simulink model "ajay"  (R2024b)
settings: Solver=ode45  StartTime=0.0  StopTime=75  RelTol=1e-3  EnableMultiTasking=on
PreLoadFcn:
  | load asbSkyHoggData.mat
StopFcn:
  | open_system('asbSkyHogg/Vehicle System Model/Avionics/Autopilot/Altitude')
model workspace (MAT data in the model file):
  LatLong0 = [45 120]
  Sref = 20.9775
  Tc = 0.0166666666667
  Thrust = 2512.574
  Ts = 0
  V0 = 93.1047999839
  alpha0 = 0.0170924
  alt0 = 2000
  beta0 = 0
  bref = 12.5425
  cbar = 1.7526
  cg_0 = [2.158 0 0]
  g_0 = [0 0 9.81]
  heading0 = 0
  inertia = [5787.969  0  117.64; 0  6928.93  0; -117.64  0  11578.329]
  mass = 1299.21378662
  maxdef_aileron = 30
  maxdef_elevator = 20
  maxdef_rudder = 60
  mindef_aileron = -30
  mindef_elevator = -20
  mindef_rudder = -60
  mpoperpoint = []
  theta0 = 0.017092
  wn_act = 44
  wy0 = 0
  z_act = 0.7
undefined symbols (not defined in the file): Earth, F, Light, MIL, pa28, statdyn, WGS84
libraries: aerolibasang x4, aerolibwind2 x3, aerolibtransform2 x3, aerolibactuator x3, aerolibatmos2 x2, aerolibconvert2 x2, aerolibadyn x2, aerolibfltsims x2, simulink x1, simulink_extras x1, aerolibnav x1, sharedtransform x1
Description:
  | Lightweight Airplane Design
  | 
  | This is the three degree-of-freedom model of a lightweight four-seater
  | low wing monoplane with a longitudinal autopilot.
settings Model: Creator=The MathWorks, Inc.  LastModifiedBy=91964
settings SolverCC: AlgebraicLoopSolver=TrustRegion  MaxZcPerStep=1
settings DataIOCC: ExternalInput=getinputstruct(op_skyhogg3dof2V5)  InitialState=getstatestruct(op_skyhogg3dof2V5)  LimitDataPoints=on  SaveFormat=Array  ReturnWorkspaceOutputs=off
settings OptimizationCC: ExpressionDepthLimit=2147483647  InitFltsAndDblsToZero=on  LifeSpan=inf
settings DebuggingCC: WriteAfterWriteMsg=DisableAll  AlgebraicLoopMsg=none  SaveWithParameterizedLinksMsg=none  SignalResolutionControl=TryResolveAllWithWarning  FcnCallInpInsideContextMsg=warning  UniqueDataStoreMsg=error  AllowSymbolicDim=off  StateNameClashWarn=warning  SubsystemReferenceDiagnosticForUnitTest=warning  StrictBusMsg=ErrorOnBusTreatedAsVector  SFUnexpectedBacktrackingDiag=warning  SFNoUnconditionalDefaultTransitionDiag=warning  SFExecutionAtInitializationDiag=none  ArithmeticOperatorsInVariantConditions=warning
settings HardwareCC: ProdBitPerPointer=32  ProdBitPerSizeT=32  ProdBitPerPtrDiffT=32  ProdLargestAtomicFloat=None  ProdIntDivRoundTo=Undefined  ProdEndianess=Unspecified  ProdWordSize=32  ProdHWDeviceType=32-bit Generic
settings ModelReferenceCC: EnableRefExpFcnMdlSchedulingChecks=on  PropagateSignalLabelsOutOfModel=off
settings SFSimCC: SimUseLocalCustomCode=off  CustomCodeUndefinedFunction=UseInterfaceOnly
settings RTWCC: RTWUseLocalCustomCode=off  GPUComputeCapability=3.5  DLArmComputeVersion=19.05
settings CodeAppCC: StateflowObjectComments=on
settings GRTTargetCC: TargetFcnLib=ansi_tfl_tmw.mat  TargetLangStandard=C89/C90 (ANSI)  CombineOutputUpdateFcns=off  GRTInterface=on
settings ConfigComp: CovMetricSettings=dw  CovSaveCumulativeToWorkspaceVar=on  CovSaveSingleToWorkspaceVar=on  CovExternalEMLEnable=off  CovSFcnEnable=off

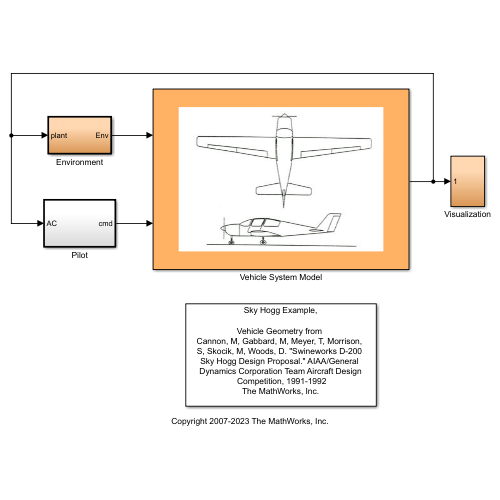
[thumbnail: Simulink's stored preview of the top-level diagram]
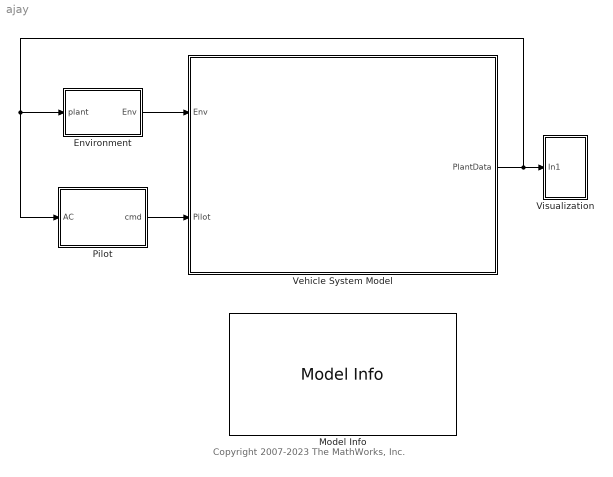
== system ajay ==
  note: Copyright 2007-2023 The MathWorks, Inc.
  Environment : Subsystem  TreatAsAtomicUnit=on
  Model Info : simulink/Model-Wide Utilities/Model Info  Frame=on  DisplayStringWithTags=|  HorizontalTextAlignment=Center  LeftAlignmentValue=0.5
      | Sky Hogg Example,
      | 
      | Vehicle Geometry from 
      | Cannon, M, Gabbard, M, Meyer, T, Morrison, 
      | S, Skocik, M, Woods, D. "Swineworks D-200 
      | Sky Hogg Design Proposal." AIAA/General 
      | Dynamics Corporation Team Aircraft Design
      |  Competition, 1991-1992
      | %<Creator>
      | %<ModifiedComment>
  Pilot : Subsystem  TreatAsAtomicUnit=on
  Vehicle System Model : Subsystem
      mask Display: image('asbSkyHogg.jpg',[.1 .1 .8 .8],'on')
  Visualization : Subsystem
  wires:
  Environment/1(Env) -> Vehicle System Model/1(Env)
  Vehicle System Model/1(PlantData) -> Environment/1(plant), Pilot/1(AC), Visualization/1(In1)
  Pilot/1(cmd) -> Vehicle System Model/2(Pilot)

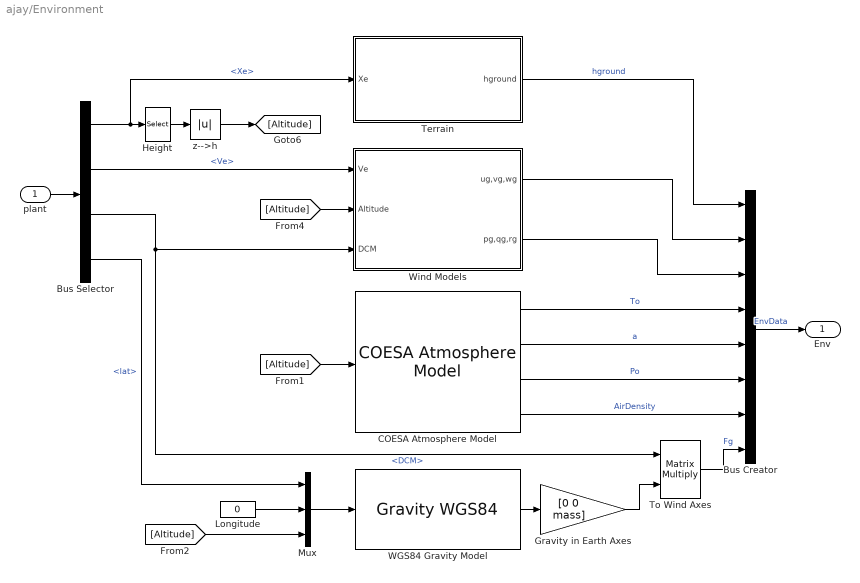
== system ajay/Environment ==
  plant : Inport
  Bus Creator : BusCreator  Inputs='hground','WindVelocity','WindAngularRates','To','a','Po','AirDensity','Fg'
  Bus Selector : BusSelector  OutputSignals=Xe,Ve,DCM,lat
  COESA Atmosphere Model : aerolibatmos2/COESA Atmosphere Model  units=Metric (MKS)  spec=1976 COESA-extended U.S. Standard Atmosphere  model=Profile  profile_var=High temperature  profile_percent=1%  profile_alt=5 km (16404 ft)  envelope_var=High temperature  envelope_percent=1%  action=Warning
  Gravity in Earth Axes : Gain  Gain=[0 0 mass]  SaturateOnIntegerOverflow=on  OutDataTypeStr=Inherit: Same as input  ParamDataTypeStr=Inherit: Same as input
  Height : Selector  IndexMode=Zero-based  InputPortWidth=3  IndexOptions=Index vector (dialog)  Indices=2  OutputSizes=1
  Longitude : Constant  Value=0
  Mux : Mux  Inputs=3
  Terrain : Subsystem
  To Wind Axes : Product  Multiplication=Matrix(*)  InputSameDT=on  SaturateOnIntegerOverflow=on  OutDataTypeStr=Inherit: Same as first input
  "WGS84 Gravity Model  " : GravityWGS84
  Wind Models : Subsystem
  z-->h : Abs
  Env : Outport  InitialOutput=0  VectorParamsAs1DForOutWhenUnconnected=off
  wires:
  Bus Selector/3 -> To Wind Axes/1, Wind Models/3(DCM)  "<DCM>"
  Bus Selector/2 -> Wind Models/1(Ve)  "<Ve>"
  Bus Selector/1 -> Height/1, Terrain/1(Xe)  "<Xe>"
  [Altitude] -> COESA Atmosphere Model/1
  [Altitude] -> Mux/3
  [Altitude] -> Wind Models/2(Altitude)
  z-->h/1 -> [Altitude]
  plant/1 -> Bus Selector/1
  Bus Creator/1 -> Env/1  "EnvData"
  To Wind Axes/1 -> Bus Creator/8  "Fg"
  Gravity in Earth Axes/1 -> To Wind Axes/2
  "WGS84 Gravity Model  "/1 -> Gravity in Earth Axes/1
  Bus Selector/4 -> Mux/1  "<lat>"
  Height/1 -> z-->h/1
  COESA Atmosphere Model/1 -> Bus Creator/4  "To"
  COESA Atmosphere Model/3 -> Bus Creator/6  "Po"
  COESA Atmosphere Model/2 -> Bus Creator/5  "a"
  COESA Atmosphere Model/4 -> Bus Creator/7  "AirDensity"
  Wind Models/2(pg,qg,rg) -> Bus Creator/3
  Wind Models/1(ug,vg,wg) -> Bus Creator/2
  Terrain/1(hground) -> Bus Creator/1  "hground"
  Mux/1 -> "WGS84 Gravity Model  "/1
  Longitude/1 -> Mux/2

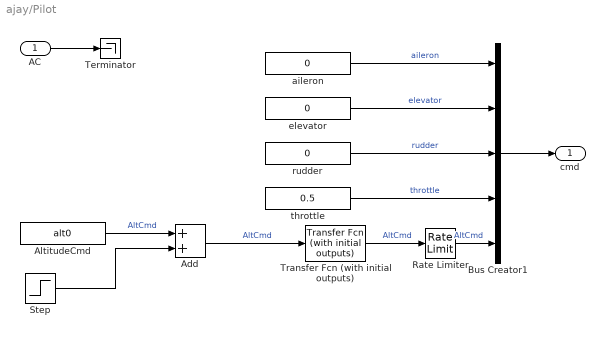
== system ajay/Pilot ==
  AC : Inport
  Add : Sum
  AltitudeCmd : Constant  Value=alt0  OutDataTypeStr=double
  Bus Creator1 : BusCreator  Inputs=5
  Rate Limiter : RateLimiter  RisingSlewLimit=500/3/60  SampleTimeMode=inherited  InitialCondition=2000
  Step : Step  Time=5  After=50  SampleTime=0
  Terminator : Terminator
  Transfer Fcn (with initial outputs) : simulink_extras/Additional Linear/Transfer Fcn (with initial outputs)  N=.25  D=[1,.25]  Y0=2000  U0=2000
  aileron : Constant  Value=0  OutDataTypeStr=single
  elevator : Constant  Value=0  OutDataTypeStr=single
  rudder : Constant  Value=0  OutDataTypeStr=single
  throttle : Constant  Value=0.5  OutDataTypeStr=double
  cmd : Outport  VectorParamsAs1DForOutWhenUnconnected=off
  wires:
  elevator/1 -> Bus Creator1/2  "elevator"
  aileron/1 -> Bus Creator1/1  "aileron"
  throttle/1 -> Bus Creator1/4  "throttle"
  rudder/1 -> Bus Creator1/3  "rudder"
  Bus Creator1/1 -> cmd/1
  AC/1 -> Terminator/1
  AltitudeCmd/1 -> Add/1  "AltCmd"
  Step/1 -> Add/2
  Add/1 -> Transfer Fcn (with initial outputs)/1  "AltCmd"
  Rate Limiter/1 -> Bus Creator1/5  "AltCmd"
  Transfer Fcn (with initial outputs)/1 -> Rate Limiter/1  "AltCmd"

== system ajay/Vehicle System Model ==
  Env : Inport
  Pilot : Inport  Port=2
  Avionics : Subsystem
  "Env " : InportShadow
  Flight Sensors : Subsystem
  "Pilot " : InportShadow  Port=2
  Vehicle : Subsystem
  PlantData : Outport  VectorParamsAs1DForOutWhenUnconnected=off
  wires:
  Env/1 -> Vehicle/1(Env)
  Vehicle/1(PlantData) -> PlantData/1, Avionics/1(PlantData), Flight Sensors/2(plant)
  Flight Sensors/1(sensed) -> Avionics/2(Sensors)
  Avionics/1(ActCmd) -> Vehicle/2(ActCmd)
  Pilot/1 -> Vehicle/3(Pilot)
  "Env "/1 -> Flight Sensors/1(Env)
  "Pilot "/1 -> Avionics/3(Pilot)

== system ajay/Visualization ==
  note: For FlightGear visualization only, we use the model for Piper Cherokee Warrior II.
  note: 3. To start FlightGear, generate run script and run generated batch file by typing
      |      dos('runfg.bat &') at the MATLAB command line.
  note: 1. See the Aerospace Blockset User's Guide for instructions to set up FlightGear.
  note: 2. Install the pa28-161 geometry model to FlightGear's data/Aircraft
      |     directory. The geometry is downloadable from www.flightgear.org.
  In1 : Inport
  Bus Selector1 : BusSelector  OutputSignals=long,lat,alt,body angles
  Bus to Vector3 : BusToVector
  FlightGear Preconfigured 6DoF Animation : aerolibfltsims/FlightGear Preconfigured 6DoF Animation  xFlightGearVersion=v2019.1  DestinationIpAddress=127.0.0.1  DestinationPort=5502  SampleTime=1/30  packetVersion=24
  Generate Run Script (if FG is installed) : aerolibfltsims/Generate Run Script  Architecture=Default  dataFlow=Send  GeometryModelName=pa28-161  AirportId=KSFO  RunwayId=10L  InitialAltitude=7224  InitialHeading=113  OffsetDistance=4.72  OffsetAzimuth=0  InstallScenery=on  DisableShaders=on  OriginAddress=127.0.0.1  DestinationPort=5502  OriginPort=5505  LocalAddress=127.0.0.1  OutputFileName=runfg.bat  FlightGearBaseDirectory=C:\Program Files\FlightGear
  Mux1 : Mux
  wires:
  In1/1 -> Bus Selector1/1
  Bus Selector1/1 -> Mux1/1  "<long>"
  Bus Selector1/2 -> Mux1/2  "<lat>"
  Bus Selector1/3 -> Mux1/3  "<alt>"
  Bus Selector1/4 -> Bus to Vector3/1  "<body angles>"
  Mux1/1 -> FlightGear Preconfigured 6DoF Animation/1
  Bus to Vector3/1 -> Mux1/4

== system ajay/Environment/Terrain ==
  note: This part of the system defines the interface for the terrain model that will be developed in detail later on.
  Xe : Inport
  Terminator : Terminator
  hground_value : Constant  Value=0  OutDataTypeStr=single
  hground : Outport  Unit=m  VectorParamsAs1DForOutWhenUnconnected=off
  wires:
  hground_value/1 -> hground/1  "hground"
  Xe/1 -> Terminator/1

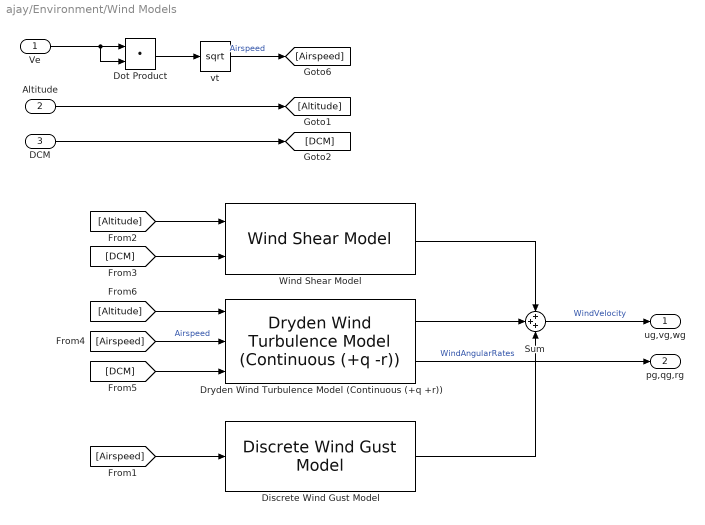
== system ajay/Environment/Wind Models ==
  Ve : Inport
  Altitude : Inport  Port=2
  DCM : Inport  Port=3
  Discrete Wind Gust Model : aerolibwind2/Discrete Wind Gust Model  units=Metric (MKS)  Gx=off  Gy=off  Gz=off  t_0=20  d_m=[120 120 80]  v_m=[3.5 3.0 3.0]
  Dot Product : DotProduct  InputSameDT=off  OutDataTypeStr=Inherit: Inherit via internal rule
  Dryden Wind Turbulence Model (Continuous (+q +r)) : aerolibwind2/Dryden Wind Turbulence Model  (Continuous (+q -r))  units=Metric (MKS)  spec=MIL-F-8785C  model=Continuous Dryden (+q +r)  W20=5  Wdeg=0  TurbProb=10^-2 - Light  L_high=533.4  Wingspan=4  ts=0.1  Seed=[23341 23342 23343 23344]  T_on=off
  Sum : Sum  Inputs=+++  InputSameDT=on  SaturateOnIntegerOverflow=on  OutDataTypeStr=Inherit: Same as first input
  Wind Shear Model : aerolibwind2/Wind Shear Model  units=Metric (MKS)  phase=Category C - Terminal Flight Phase  W_20=1  Wdeg=0
  vt : Sqrt
  ug,vg,wg : Outport  Unit=m/s  VectorParamsAs1DForOutWhenUnconnected=off
  pg,qg,rg : Outport  Port=2  Unit=rad/second  VectorParamsAs1DForOutWhenUnconnected=off
  wires:
  [Altitude] -> Dryden Wind Turbulence Model (Continuous (+q +r))/1
  [DCM] -> Dryden Wind Turbulence Model (Continuous (+q +r))/3
  [DCM] -> Wind Shear Model/2
  DCM/1 -> [DCM]
  [Altitude] -> Wind Shear Model/1
  Altitude/1 -> [Altitude]
  [Airspeed] -> Discrete Wind Gust Model/1
  vt/1 -> [Airspeed]  "Airspeed"
  Dot Product/1 -> vt/1
  Dryden Wind Turbulence Model (Continuous (+q +r))/2 -> pg,qg,rg/1  "WindAngularRates"
  [Airspeed] -> Dryden Wind Turbulence Model (Continuous (+q +r))/2  "Airspeed"
  Sum/1 -> ug,vg,wg/1  "WindVelocity"
  Discrete Wind Gust Model/1 -> Sum/3
  Dryden Wind Turbulence Model (Continuous (+q +r))/1 -> Sum/2
  Wind Shear Model/1 -> Sum/1
  Ve/1 -> Dot Product/2, Dot Product/1

== system ajay/Vehicle System Model/Avionics ==
  PlantData : Inport
  Sensors : Inport  Port=2
  Pilot : Inport  Port=3
  Air Data Computer : Subsystem  TreatAsAtomicUnit=on
  Autopilot : Subsystem
  Bus Creator : BusCreator  Inputs=2
  Bus Selector1 : BusSelector  OutputSignals=Ab,w,wdot
  Center of Gravity : Constant  Value=cg_0  SampleTime=Tc
  Gravity (not in Accels) : Constant  Value=g_0  SampleTime=Tc
  Guidance : Subsystem
  Three-axis IMU : aerolibnav/Three-axis Inertial Measurement Unit  units=Metric (MKS)  imu=cg_0  i_Ts=Tc  dtype_a=off  w_a=190  z_a=0.707  a_sf_cc=[1 0 0; 0 1 0; 0 0 1]  a_bias=[0 0 0]  a_sat="[-inf  -inf  -inf  inf inf inf]"  dtype_g=off  w_g=190  z_g=0.707  g_sf_cc=[1 0 0; 0 1 0; 0 0 1]  g_bias=[0 0 0]  g_sens=[0 0 0]  g_sat="[-inf  -inf  -inf  inf inf inf]"  i_rand=off  i_seeds=[23093 23094 23095 23096 23097 23098]  i_pow=[0.001 0.001 0.001 0.0001 0.0001 0.0001]
  ActCmd : Outport  VectorParamsAs1DForOutWhenUnconnected=off
  wires:
  Three-axis IMU/2 -> Bus Creator/2
  Three-axis IMU/1 -> Bus Creator/1
  Bus Selector1/1 -> Three-axis IMU/1  "<Ab>"
  Center of Gravity/1 -> Three-axis IMU/4
  Bus Creator/1 -> Autopilot/1(AvionicBus), Guidance/2(AvionicBus)
  PlantData/1 -> Bus Selector1/1
  Bus Selector1/2 -> Three-axis IMU/2  "<w>"
  Bus Selector1/3 -> Three-axis IMU/3  "<wdot>"
  Gravity (not in Accels)/1 -> Three-axis IMU/5
  Sensors/1 -> Air Data Computer/1(sensors)
  Autopilot/1(cmd) -> ActCmd/1
  Air Data Computer/1(AirData) -> Autopilot/2(AirData), Guidance/1(AirData)
  Guidance/1(cmd) -> Autopilot/3(guidance)
  Pilot/1 -> Guidance/3(Pilot)

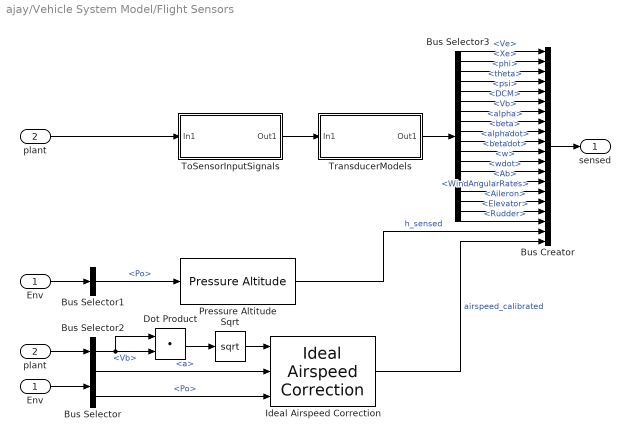
== system ajay/Vehicle System Model/Flight Sensors ==
  Env : Inport
  plant : Inport  Port=2
  Bus Creator : BusCreator  Inputs=20
  Bus Selector : BusSelector  OutputSignals=a,Po
  Bus Selector1 : BusSelector  OutputSignals=Po
  Bus Selector2 : BusSelector  OutputSignals=Vb
  Bus Selector3 : BusSelector  OutputSignals=Ve,Xe,body angles.phi,body angles.theta,body angles.psi,DCM,Vb,alpha,beta,alphadot,betadot,w,wdot,Ab,WindAngularRates,Act_positions.Aileron,Act_positions.Elevator,Act_positions.Rudder
  Dot Product : DotProduct  OutDataTypeStr=Inherit: Inherit via internal rule
  "Env " : InportShadow
  Ideal Airspeed Correction : aerolibasang/Ideal Airspeed Correction  units=Metric (MKS)  vel_in=TAS  vel_out_tas=CAS  vel_out_eas=CAS  vel_out_cas=TAS  method=Table Lookup  SubOnly=off  action=Error
  Pressure Altitude : aerolibatmos2/Pressure Altitude  units=Metric (MKS)  action=Warning
  Sqrt : Sqrt
  ToSensorInputSignals : Subsystem
  TransducerModels : Subsystem
  "plant " : InportShadow  Port=2
  sensed : Outport  VectorParamsAs1DForOutWhenUnconnected=off
  wires:
  ToSensorInputSignals/1(Out1) -> TransducerModels/1(In1)
  Env/1 -> Bus Selector/1
  TransducerModels/1(Out1) -> Bus Selector3/1
  plant/1 -> ToSensorInputSignals/1(In1)
  Bus Selector/1 -> Ideal Airspeed Correction/2  "<a>"
  Bus Selector/2 -> Ideal Airspeed Correction/3  "<Po>"
  Bus Selector1/1 -> Pressure Altitude/1  "<Po>"
  "Env "/1 -> Bus Selector1/1
  "plant "/1 -> Bus Selector2/1
  Dot Product/1 -> Sqrt/1
  Sqrt/1 -> Ideal Airspeed Correction/1
  Bus Selector2/1 -> Dot Product/2, Dot Product/1  "<Vb>"
  Bus Selector3/1 -> Bus Creator/1  "<Ve>"
  Bus Selector3/2 -> Bus Creator/2  "<Xe>"
  Bus Selector3/3 -> Bus Creator/3  "<phi>"
  Bus Selector3/4 -> Bus Creator/4  "<theta>"
  Bus Selector3/5 -> Bus Creator/5  "<psi>"
  Bus Selector3/6 -> Bus Creator/6  "<DCM>"
  Bus Selector3/7 -> Bus Creator/7  "<Vb>"
  Bus Selector3/8 -> Bus Creator/8  "<alpha>"
  Bus Selector3/9 -> Bus Creator/9  "<beta>"
  Bus Selector3/10 -> Bus Creator/10  "<alphadot>"
  Bus Selector3/11 -> Bus Creator/11  "<betadot>"
  Bus Selector3/12 -> Bus Creator/12  "<w>"
  Bus Selector3/13 -> Bus Creator/13  "<wdot>"
  Bus Selector3/14 -> Bus Creator/14  "<Ab>"
  Bus Creator/1 -> sensed/1
  Bus Selector3/15 -> Bus Creator/15  "<WindAngularRates>"
  Bus Selector3/16 -> Bus Creator/16  "<Aileron>"
  Bus Selector3/17 -> Bus Creator/17  "<Elevator>"
  Bus Selector3/18 -> Bus Creator/18  "<Rudder>"
  Pressure Altitude/1 -> Bus Creator/19  "h_sensed"
  Ideal Airspeed Correction/1 -> Bus Creator/20  "airspeed_calibrated"

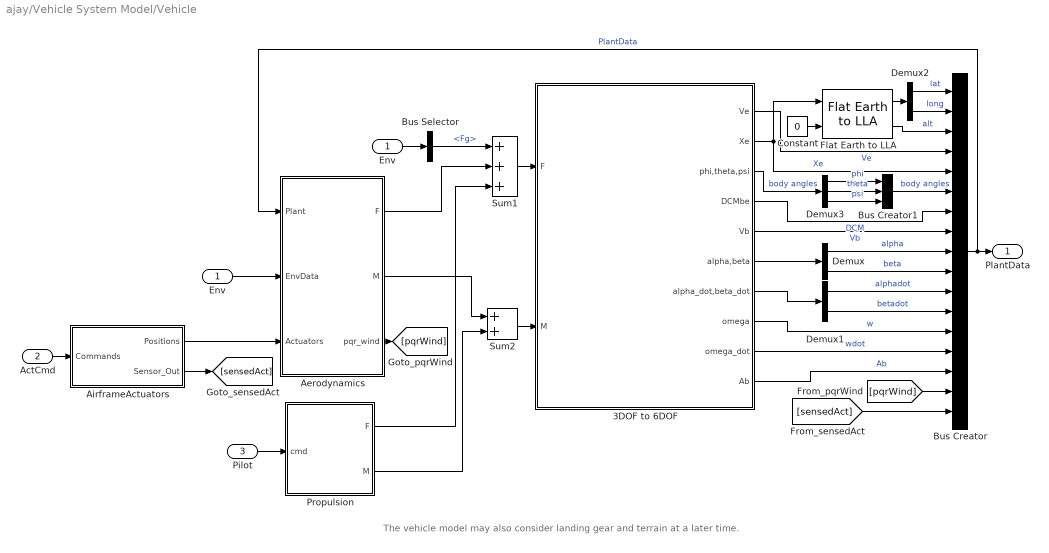
== system ajay/Vehicle System Model/Vehicle ==
  note: The vehicle model may also consider landing gear and terrain at a later time.
  Env : Inport
  ActCmd : Inport  Port=2
  Pilot : Inport  Port=3
  3DOF to 6DOF : Subsystem
  Aerodynamics : Subsystem
  AirframeActuators : Subsystem
  Bus Creator : BusCreator  Inputs=17
  Bus Creator1 : BusCreator  Inputs=3
  Bus Selector : BusSelector  OutputSignals=Fg
  Constant : Constant  Value=0
  Demux : Demux  Outputs=2
  Demux1 : Demux  Outputs=2
  Demux2 : Demux  Outputs=2
  Demux3 : Demux  Outputs=3
  "Env " : InportShadow
  Flat Earth to LLA : aerolibtransform2/Flat Earth to LLA  units=Metric (MKS)  ptype=Earth (WGS84)  F=1/298.257223563  R=6378137  refPosPort=off  LL0=LatLong0  psi=heading0
  Propulsion : Subsystem
      settings: RTWSystemCode=Inline
  Sum1 : Sum  Inputs=+++  InputSameDT=on  SaturateOnIntegerOverflow=on  OutDataTypeStr=Inherit: Same as first input
  Sum2 : Sum  InputSameDT=on  SaturateOnIntegerOverflow=on  OutDataTypeStr=Inherit: Same as first input
  PlantData : Outport  VectorParamsAs1DForOutWhenUnconnected=off
  wires:
  Sum1/1 -> 3DOF to 6DOF/1(F)
  Sum2/1 -> 3DOF to 6DOF/2(M)
  3DOF to 6DOF/3(phi,theta,psi) -> Demux3/1  "body angles"
  3DOF to 6DOF/4(DCMbe) -> Bus Creator/7  "DCM"
  3DOF to 6DOF/5(Vb) -> Bus Creator/8  "Vb"
  3DOF to 6DOF/6(alpha,beta) -> Demux/1
  3DOF to 6DOF/7(alpha_dot,beta_dot) -> Demux1/1
  3DOF to 6DOF/9(omega_dot) -> Bus Creator/14  "wdot"
  3DOF to 6DOF/10(Ab) -> Bus Creator/15  "Ab"
  Aerodynamics/1(F) -> Sum1/2
  Aerodynamics/2(M) -> Sum2/1
  Propulsion/1(F) -> Sum1/3
  Propulsion/2(M) -> Sum2/2
  Bus Selector/1 -> Sum1/1  "<Fg>"
  Env/1 -> Aerodynamics/2(EnvData)
  ActCmd/1 -> AirframeActuators/1(Commands)
  Pilot/1 -> Propulsion/1(cmd)
  "Env "/1 -> Bus Selector/1
  AirframeActuators/1(Positions) -> Aerodynamics/3(Actuators)
  Aerodynamics/3(pqr_wind) -> [pqrWind]
  [pqrWind] -> Bus Creator/16
  AirframeActuators/2(Sensor_Out) -> [sensedAct]
  [sensedAct] -> Bus Creator/17
  Constant/1 -> Flat Earth to LLA/2
  Flat Earth to LLA/2 -> Bus Creator/3  "alt"
  Flat Earth to LLA/1 -> Demux2/1
  Demux2/1 -> Bus Creator/1  "lat"
  Demux2/2 -> Bus Creator/2  "long"
  Demux1/1 -> Bus Creator/11  "alphadot"
  Demux1/2 -> Bus Creator/12  "betadot"
  Demux3/1 -> Bus Creator1/1  "phi"
  Demux3/2 -> Bus Creator1/2  "theta"
  Demux3/3 -> Bus Creator1/3  "psi"
  Bus Creator1/1 -> Bus Creator/6  "body angles"
  3DOF to 6DOF/8(omega) -> Bus Creator/13  "w"
  Demux/2 -> Bus Creator/10  "beta"
  Demux/1 -> Bus Creator/9  "alpha"
  3DOF to 6DOF/1(Ve) -> Bus Creator/4  "Ve"
  3DOF to 6DOF/2(Xe) -> Flat Earth to LLA/1, Bus Creator/5  "Xe"
  Bus Creator/1 -> Aerodynamics/1(Plant), PlantData/1  "PlantData"

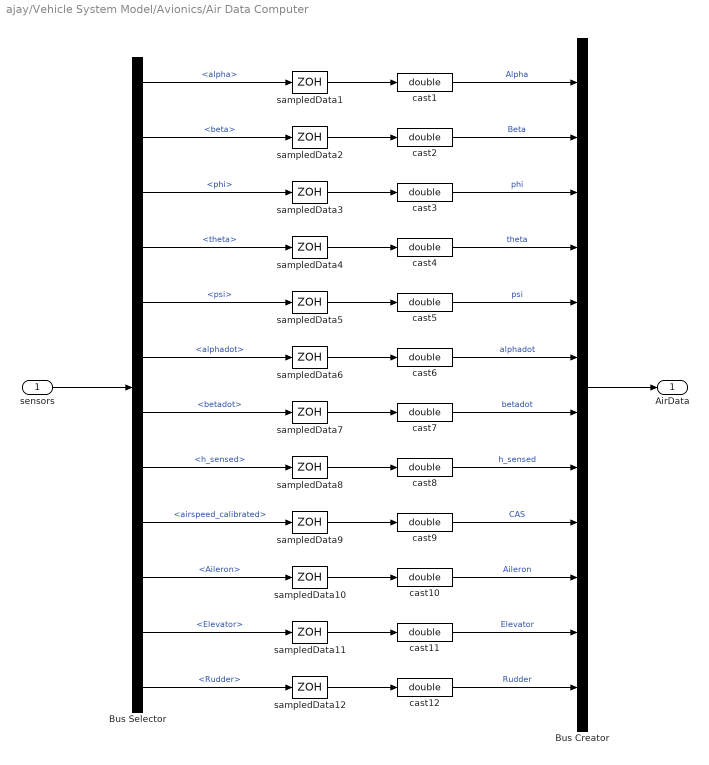
== system ajay/Vehicle System Model/Avionics/Air Data Computer ==
  sensors : Inport  SampleTime=Ts
  Bus Creator : BusCreator  Inputs=12
  Bus Selector : BusSelector  OutputSignals=alpha,beta,phi,theta,psi,alphadot,betadot,h_sensed,airspeed_calibrated,Aileron,Elevator,Rudder
  cast{1..12} (12 alike) : DataTypeConversion  OutDataTypeStr=double  SaturateOnIntegerOverflow=off  RndMeth=Floor
  sampledData{1..12} (12 alike) : ZeroOrderHold  SampleTime=Tc
  AirData : Outport  VectorParamsAs1DForOutWhenUnconnected=off
  wires:
  sensors/1 -> Bus Selector/1
  Bus Creator/1 -> AirData/1
  cast1/1 -> Bus Creator/1  "Alpha"
  cast2/1 -> Bus Creator/2  "Beta"
  cast3/1 -> Bus Creator/3  "phi"
  cast12/1 -> Bus Creator/12  "Rudder"
  cast10/1 -> Bus Creator/10  "Aileron"
  cast9/1 -> Bus Creator/9  "CAS"
  cast8/1 -> Bus Creator/8  "h_sensed"
  cast7/1 -> Bus Creator/7  "betadot"
  cast6/1 -> Bus Creator/6  "alphadot"
  cast5/1 -> Bus Creator/5  "psi"
  sampledData1/1 -> cast1/1
  sampledData2/1 -> cast2/1
  sampledData3/1 -> cast3/1
  sampledData4/1 -> cast4/1
  sampledData5/1 -> cast5/1
  sampledData6/1 -> cast6/1
  sampledData7/1 -> cast7/1
  sampledData8/1 -> cast8/1
  sampledData9/1 -> cast9/1
  sampledData10/1 -> cast10/1
  cast4/1 -> Bus Creator/4  "theta"
  Bus Selector/1 -> sampledData1/1  "<alpha>"
  Bus Selector/2 -> sampledData2/1  "<beta>"
  Bus Selector/3 -> sampledData3/1  "<phi>"
  Bus Selector/4 -> sampledData4/1  "<theta>"
  Bus Selector/5 -> sampledData5/1  "<psi>"
  Bus Selector/6 -> sampledData6/1  "<alphadot>"
  Bus Selector/7 -> sampledData7/1  "<betadot>"
  Bus Selector/8 -> sampledData8/1  "<h_sensed>"
  Bus Selector/9 -> sampledData9/1  "<airspeed_calibrated>"
  Bus Selector/10 -> sampledData10/1  "<Aileron>"
  Bus Selector/12 -> sampledData12/1  "<Rudder>"
  sampledData11/1 -> cast11/1
  sampledData12/1 -> cast12/1
  Bus Selector/11 -> sampledData11/1  "<Elevator>"
  cast11/1 -> Bus Creator/11  "Elevator"

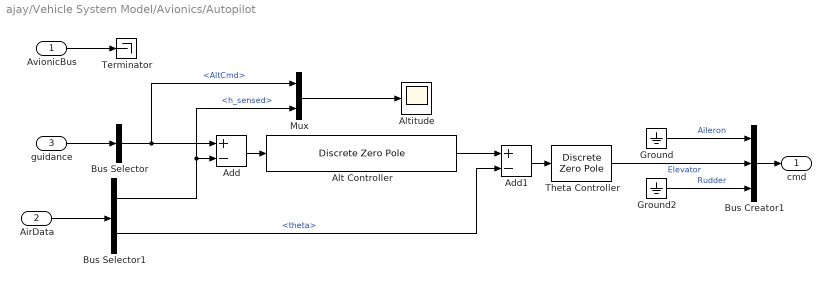
== system ajay/Vehicle System Model/Avionics/Autopilot ==
  AvionicBus : Inport
  AirData : Inport  Port=2
  guidance : Inport  Port=3
  Add : Sum  Inputs=+-
  Add1 : Sum  Inputs=+-
  Alt Controller : DiscreteZeroPole  Zeros=[0.998853192323097;0.977076159863424]  Poles=[1;0.920841826994512]  Gain=0.0337283240400683  SampleTime=Tc
  Altitude : Scope
  Bus Creator1 : BusCreator  Inputs=3
  Bus Selector : BusSelector  OutputSignals=AltCmd
  Bus Selector1 : BusSelector  OutputSignals=h_sensed,theta
  Ground : Ground
  Ground2 : Ground
  Mux : Mux  Inputs=2
  Terminator : Terminator
  Theta Controller : DiscreteZeroPole  Zeros=0.999268009521977  Poles=1  Gain=-261.8699347622  SampleTime=Tc
  cmd : Outport  VectorParamsAs1DForOutWhenUnconnected=off
  wires:
  Add1/1 -> Theta Controller/1
  Alt Controller/1 -> Add1/1
  Add/1 -> Alt Controller/1
  Bus Selector/1 -> Mux/1, Add/1  "<AltCmd>"
  guidance/1 -> Bus Selector/1
  AirData/1 -> Bus Selector1/1
  AvionicBus/1 -> Terminator/1
  Bus Creator1/1 -> cmd/1
  Ground2/1 -> Bus Creator1/3  "Rudder"
  Theta Controller/1 -> Bus Creator1/2  "Elevator"
  Ground/1 -> Bus Creator1/1  "Aileron"
  Mux/1 -> Altitude/1
  Bus Selector1/1 -> Mux/2, Add/2  "<h_sensed>"
  Bus Selector1/2 -> Add1/2  "<theta>"

== system ajay/Vehicle System Model/Avionics/Guidance ==
  note: This part of the system defines the interface for the guidance model that will be developed in detail later on.
  AirData : Inport
  AvionicBus : Inport  Port=2
  Pilot : Inport  Port=3
  Bus Creator1 : BusCreator  Inputs=2
  Bus Selector : BusSelector  OutputSignals=AltCmd
  Ground1 : Ground
  Terminator : Terminator
  Terminator1 : Terminator
  cmd : Outport  VectorParamsAs1DForOutWhenUnconnected=off
  wires:
  Pilot/1 -> Bus Selector/1
  Bus Selector/1 -> Bus Creator1/1  "<AltCmd>"
  Ground1/1 -> Bus Creator1/2  "Elevator angle"
  Bus Creator1/1 -> cmd/1
  AvionicBus/1 -> Terminator/1
  AirData/1 -> Terminator1/1

== system ajay/Vehicle System Model/Flight Sensors/ToSensorInputSignals ==
  note: This part of the system defines the interface for the measurement noise model that
      |  will be developed in detail later on.
  In1 : Inport
  Out1 : Outport  VectorParamsAs1DForOutWhenUnconnected=off
  wires:
  In1/1 -> Out1/1

== system ajay/Vehicle System Model/Flight Sensors/TransducerModels ==
  note: This part of the system defines the interface for the transducers model that
      |  will be developed in detail later on.
  In1 : Inport
  Out1 : Outport  VectorParamsAs1DForOutWhenUnconnected=off
  wires:
  In1/1 -> Out1/1

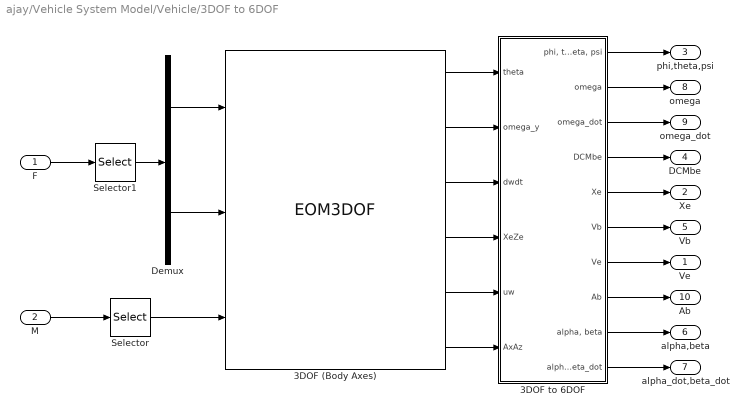
== system ajay/Vehicle System Model/Vehicle/3DOF to 6DOF ==
  F : Inport
  M : Inport  Port=2
  3DOF (Body Axes) : EOM3DOF  v_ini=V0  theta_ini=theta0  q_ini=wy0  alpha_ini=alpha0  pos_ini=[0 -alt0]  mass=mass  Iyy=inertia(2,2)  g=0  mdot_flag=off
  3DOF to 6DOF : Subsystem
  Demux : Demux  Outputs=2
  Selector : Selector  IndexMode=Zero-based  InputPortWidth=3  IndexOptions=Index vector (dialog)  Indices=1  OutputSizes=1
  Selector1 : Selector  IndexMode=Zero-based  InputPortWidth=3  IndexOptions=Index vector (dialog)  Indices=[0 2]  OutputSizes=1
  Ve : Outport  Unit=m/s  VectorParamsAs1DForOutWhenUnconnected=off
  Xe : Outport  Port=2  Unit=m  VectorParamsAs1DForOutWhenUnconnected=off
  phi,theta,psi : Outport  Port=3  Unit=rad  VectorParamsAs1DForOutWhenUnconnected=off
  DCMbe : Outport  Port=4  VectorParamsAs1DForOutWhenUnconnected=off
  Vb : Outport  Port=5  Unit=m/s  VectorParamsAs1DForOutWhenUnconnected=off
  alpha,beta : Outport  Port=6  Unit=rad  VectorParamsAs1DForOutWhenUnconnected=off
  alpha_dot,beta_dot : Outport  Port=7  Unit=rad/s  VectorParamsAs1DForOutWhenUnconnected=off
  omega : Outport  Port=8  Unit=rad/s  VectorParamsAs1DForOutWhenUnconnected=off
  omega_dot : Outport  Port=9  Unit=rad/s^2  VectorParamsAs1DForOutWhenUnconnected=off
  Ab : Outport  Port=10  Unit=m/s^2  VectorParamsAs1DForOutWhenUnconnected=off
  wires:
  3DOF (Body Axes)/1 -> 3DOF to 6DOF/1(theta)
  Selector/1 -> 3DOF (Body Axes)/3
  Selector1/1 -> Demux/1
  3DOF to 6DOF/2(omega) -> omega/1
  3DOF to 6DOF/3(omega_dot) -> omega_dot/1
  3DOF to 6DOF/5(Xe) -> Xe/1
  3DOF to 6DOF/7(Ve) -> Ve/1
  3DOF to 6DOF/10("alpha_dot, beta_dot") -> alpha_dot,beta_dot/1
  3DOF to 6DOF/1("phi, theta, psi") -> phi,theta,psi/1
  3DOF (Body Axes)/2 -> 3DOF to 6DOF/2(omega_y)
  3DOF to 6DOF/6(Vb) -> Vb/1
  3DOF to 6DOF/8(Ab) -> Ab/1
  3DOF to 6DOF/9("alpha, beta") -> alpha,beta/1
  3DOF to 6DOF/4(DCMbe) -> DCMbe/1
  3DOF (Body Axes)/3 -> 3DOF to 6DOF/3(dwdt)
  3DOF (Body Axes)/4 -> 3DOF to 6DOF/4(XeZe)
  3DOF (Body Axes)/5 -> 3DOF to 6DOF/5(uw)
  3DOF (Body Axes)/6 -> 3DOF to 6DOF/6(AxAz)
  Demux/1 -> 3DOF (Body Axes)/1
  Demux/2 -> 3DOF (Body Axes)/2
  F/1 -> Selector1/1
  M/1 -> Selector/1

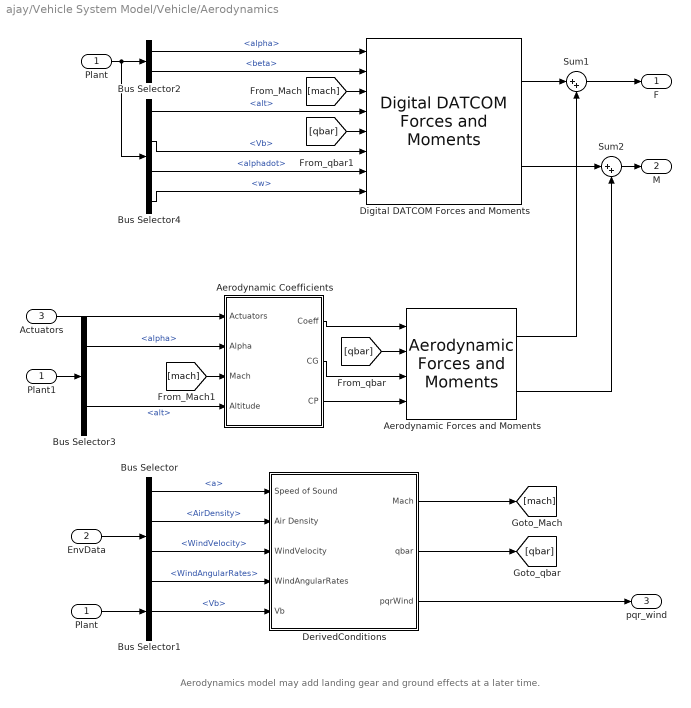
== system ajay/Vehicle System Model/Vehicle/Aerodynamics ==
  note: Aerodynamics model may add landing gear and ground effects at a later time.
  Plant : Inport
  EnvData : Inport  Port=2
  Actuators : Inport  Port=3
  Aerodynamic Coefficients : Subsystem
  "Aerodynamic Forces and Moments " : aerolibadyn/Aerodynamic Forces and Moments   inputAxes=Body  outputForceAxes=Body  outputMomentAxes=Body  S=Sref  b=bref  cbar=cbar
  Bus Selector : BusSelector  OutputSignals=a,AirDensity,WindVelocity,WindAngularRates
  Bus Selector1 : BusSelector  OutputSignals=Vb
  Bus Selector2 : BusSelector  OutputSignals=alpha,beta
  Bus Selector3 : BusSelector  OutputSignals=alpha,alt
  Bus Selector4 : BusSelector  OutputSignals=alt,Vb,alphadot,w
  DerivedConditions : Subsystem
  Digital DATCOM Forces and Moments : aerolibadyn/Digital DATCOM Forces and Moments  units=Metric (MKS)  dcase=statdyn{1}  fmode=Body  buildno=0  imethod=Linear  emethod=Linear  rmethod=Linear Extrapolation  action=None
  "Plant " : InportShadow
  Plant1 : InportShadow
  Sum1 : Sum  Inputs=|++
  Sum2 : Sum  Inputs=|++
  F : Outport  Unit=N  VectorParamsAs1DForOutWhenUnconnected=off
  M : Outport  Port=2  Unit=N*m  VectorParamsAs1DForOutWhenUnconnected=off
  pqr_wind : Outport  Port=3  Unit=rad/s  VectorParamsAs1DForOutWhenUnconnected=off
  wires:
  Digital DATCOM Forces and Moments/1 -> Sum1/1
  Digital DATCOM Forces and Moments/2 -> Sum2/1
  Aerodynamic Coefficients/1(Coeff) -> "Aerodynamic Forces and Moments "/1
  Sum1/1 -> F/1
  "Aerodynamic Forces and Moments "/1 -> Sum1/2
  Sum2/1 -> M/1
  "Aerodynamic Forces and Moments "/2 -> Sum2/2
  EnvData/1 -> Bus Selector/1
  Bus Selector/1 -> DerivedConditions/1(Speed of Sound)  "<a>"
  Bus Selector/2 -> DerivedConditions/2(Air Density)  "<AirDensity>"
  Bus Selector/3 -> DerivedConditions/3(WindVelocity)  "<WindVelocity>"
  Bus Selector/4 -> DerivedConditions/4(WindAngularRates)  "<WindAngularRates>"
  "Plant "/1 -> Bus Selector1/1
  Bus Selector1/1 -> DerivedConditions/5(Vb)  "<Vb>"
  Plant/1 -> Bus Selector2/1, Bus Selector4/1
  Bus Selector2/1 -> Digital DATCOM Forces and Moments/1  "<alpha>"
  Bus Selector2/2 -> Digital DATCOM Forces and Moments/2  "<beta>"
  Plant1/1 -> Bus Selector3/1
  Bus Selector3/1 -> Aerodynamic Coefficients/2(Alpha)  "<alpha>"
  DerivedConditions/1(Mach) -> [mach]
  [mach] -> Digital DATCOM Forces and Moments/3
  Aerodynamic Coefficients/2(CG) -> "Aerodynamic Forces and Moments "/3
  Aerodynamic Coefficients/3(CP) -> "Aerodynamic Forces and Moments "/4
  DerivedConditions/2(qbar) -> [qbar]
  [qbar] -> "Aerodynamic Forces and Moments "/2
  [qbar] -> Digital DATCOM Forces and Moments/5
  Bus Selector4/2 -> Digital DATCOM Forces and Moments/6  "<Vb>"
  Bus Selector4/1 -> Digital DATCOM Forces and Moments/4  "<alt>"
  DerivedConditions/3("pqrWind ") -> pqr_wind/1
  Bus Selector4/3 -> Digital DATCOM Forces and Moments/7  "<alphadot>"
  Bus Selector4/4 -> Digital DATCOM Forces and Moments/8  "<w>"
  Actuators/1 -> Aerodynamic Coefficients/1(Actuators)
  Bus Selector3/2 -> Aerodynamic Coefficients/4(Altitude)  "<alt>"
  [mach] -> Aerodynamic Coefficients/3(Mach)

== system ajay/Vehicle System Model/Vehicle/AirframeActuators ==
  Commands : Inport
  Bus Creator : BusCreator  Inputs=3
  Bus Selector1 : BusSelector  OutputSignals=Aileron,Elevator,Rudder
  Nonlinear Second-Order Actuator : aerolibactuator/Nonlinear Second-Order Actuator  wn_fin=wn_act  z_fin=z_act  fin_max=maxdef_aileron  fin_min=mindef_aileron  fin_maxrate=Inf  fin_act_0=0  fin_act_vel=0
  Nonlinear Second-Order Actuator1 : aerolibactuator/Nonlinear Second-Order Actuator  wn_fin=wn_act  z_fin=z_act  fin_max=maxdef_elevator  fin_min=mindef_elevator  fin_maxrate=Inf  fin_act_0=0  fin_act_vel=0
  Nonlinear Second-Order Actuator2 : aerolibactuator/Nonlinear Second-Order Actuator  wn_fin=wn_act  z_fin=z_act  fin_max=maxdef_rudder  fin_min=mindef_rudder  fin_maxrate=Inf  fin_act_0=0  fin_act_vel=0
  Positions : Outport  VectorParamsAs1DForOutWhenUnconnected=off
  Sensor_Out : Outport  Port=2  VectorParamsAs1DForOutWhenUnconnected=off
  wires:
  Commands/1 -> Bus Selector1/1
  Bus Selector1/1 -> Nonlinear Second-Order Actuator/1  "<Aileron>"
  Bus Selector1/2 -> Nonlinear Second-Order Actuator1/1  "<Elevator>"
  Bus Selector1/3 -> Nonlinear Second-Order Actuator2/1  "<Rudder>"
  Nonlinear Second-Order Actuator2/1 -> Bus Creator/3  "Rudder"
  Bus Creator/1 -> Sensor_Out/1, Positions/1  "Act_positions"
  Nonlinear Second-Order Actuator/1 -> Bus Creator/1  "Aileron"
  Nonlinear Second-Order Actuator1/1 -> Bus Creator/2  "Elevator"

== system ajay/Vehicle System Model/Vehicle/Propulsion ==
  cmd : Inport  SampleTime=Ts
  Bus Selector2 : BusSelector  OutputSignals=throttle
  Mux : Mux  Inputs=[1 2]
  ThrustX : Lookup_n-D  NumberOfTableDimensions=1  LookupTableObject=''  BreakpointsForDimension1=(1/6)*(3+([-3:3]))  IndexSearchMethod=Linear search  BeginIndexSearchUsingPreviousIndexResult=on  Table=Thrust*(1+tanh([-3:3]))  ExtrapMethod=Clip
  Thrust_LMN : Constant  Value=[0, 0, 0]  SampleTime=Ts
  Thrust_YZ : Constant  Value=[0, 0]  SampleTime=Ts
  F : Outport  Unit=N  VectorParamsAs1DForOutWhenUnconnected=off
  M : Outport  Port=2  Unit=N*m  VectorParamsAs1DForOutWhenUnconnected=off
  wires:
  ThrustX/1 -> Mux/1
  Thrust_YZ/1 -> Mux/2
  Mux/1 -> F/1
  cmd/1 -> Bus Selector2/1
  Thrust_LMN/1 -> M/1
  Bus Selector2/1 -> ThrustX/1  "<throttle>"

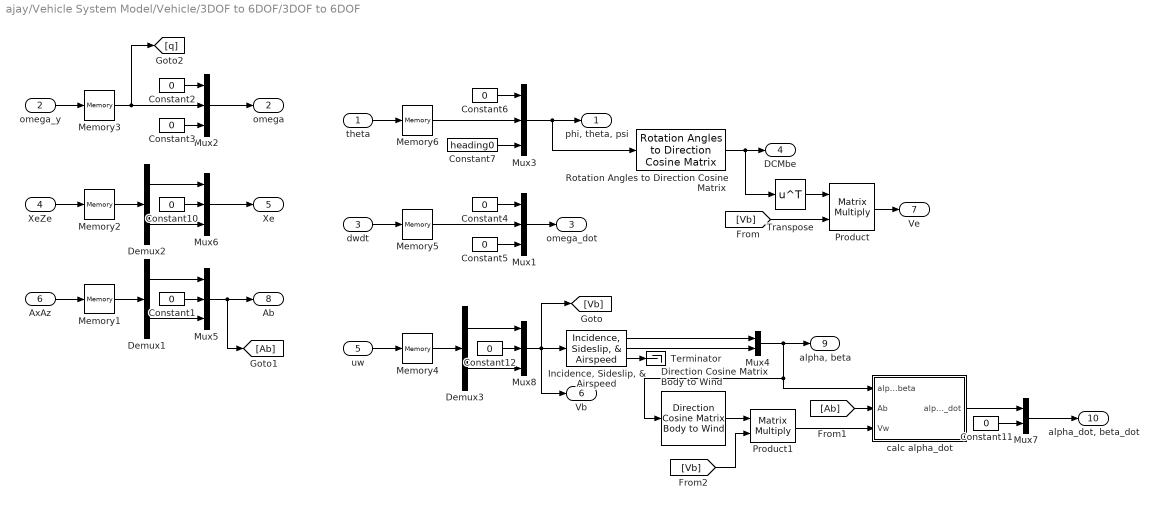
== system ajay/Vehicle System Model/Vehicle/3DOF to 6DOF/3DOF to 6DOF ==
  theta : Inport
  omega_y : Inport  Port=2
  dwdt : Inport  Port=3
  XeZe : Inport  Port=4
  uw : Inport  Port=5
  AxAz : Inport  Port=6
  Constant{1..6,10..12} (9 alike) : Constant  Value=0
  Constant7 : Constant  Value=heading0
  Demux1 : Demux  Outputs=2
  Demux2 : Demux  Outputs=2
  Demux3 : Demux  Outputs=2
  Direction Cosine Matrix Body to Wind : aerolibtransform2/Direction Cosine Matrix Body to Wind
  "Incidence, Sideslip, & Airspeed" : aerolibasang/Incidence, Sideslip, & Airspeed
  Memory1 : Memory
  Memory2 : Memory  InitialCondition=[0 -alt0]
  Memory3 : Memory  InitialCondition=wy0
  Memory4 : Memory  InitialCondition=[V0 0]
  Memory5 : Memory
  Memory6 : Memory  InitialCondition=theta0
  Mux{1..3,5..6,8} (6 alike) : Mux  Inputs=3
  Mux4 : Mux  Inputs=2
  Mux7 : Mux  Inputs=2
  Product : Product  Multiplication=Matrix(*)  InputSameDT=on  SaturateOnIntegerOverflow=on  OutDataTypeStr=Inherit: Same as first input
  Product1 : Product  Multiplication=Matrix(*)  InputSameDT=on  SaturateOnIntegerOverflow=on  OutDataTypeStr=Inherit: Same as first input
  Rotation Angles to Direction Cosine Matrix : sharedtransform/Rotation Angles to Direction Cosine Matrix  rotationOrder=ZYX  aMode=aMode
  Terminator : Terminator
  Transpose : Math  Operator=transpose  SignedPower=on
  calc alpha_dot : Subsystem
  "phi, theta, psi" : Outport  Unit=rad  VectorParamsAs1DForOutWhenUnconnected=off
  omega : Outport  Port=2  Unit=rad/s  VectorParamsAs1DForOutWhenUnconnected=off
  omega_dot : Outport  Port=3  Unit=rad/s^2  VectorParamsAs1DForOutWhenUnconnected=off
  DCMbe : Outport  Port=4  VectorParamsAs1DForOutWhenUnconnected=off
  Xe : Outport  Port=5  Unit=m  VectorParamsAs1DForOutWhenUnconnected=off
  Vb : Outport  Port=6  Unit=m/s  VectorParamsAs1DForOutWhenUnconnected=off
  Ve : Outport  Port=7  Unit=m/s  VectorParamsAs1DForOutWhenUnconnected=off
  Ab : Outport  Port=8  Unit=m/s^2  VectorParamsAs1DForOutWhenUnconnected=off
  "alpha, beta" : Outport  Port=9  Unit=rad  VectorParamsAs1DForOutWhenUnconnected=off
  "alpha_dot, beta_dot" : Outport  Port=10  Unit=rad/s  VectorParamsAs1DForOutWhenUnconnected=off
  wires:
  Mux5/1 -> Ab/1, [Ab]
  Demux1/1 -> Mux5/1
  Demux1/2 -> Mux5/3
  Constant1/1 -> Mux5/2
  Constant2/1 -> Mux2/1
  Constant3/1 -> Mux2/3
  Constant4/1 -> Mux1/1
  Constant6/1 -> Mux3/1
  Constant7/1 -> Mux3/3
  Mux3/1 -> "phi, theta, psi"/1, Rotation Angles to Direction Cosine Matrix/1
  Mux4/1 -> "alpha, beta"/1, Direction Cosine Matrix Body to Wind/1, calc alpha_dot/1(alpha,beta)
  "Incidence, Sideslip, & Airspeed"/2 -> Mux4/2
  Demux2/1 -> Mux6/1
  Demux2/2 -> Mux6/3
  Constant10/1 -> Mux6/2
  Transpose/1 -> Product/1
  [Vb] -> Product/2
  calc alpha_dot/1(alpha_dot) -> Mux7/1
  [Ab] -> calc alpha_dot/2(Ab)
  [Vb] -> Product1/2
  Constant11/1 -> Mux7/2
  Demux3/2 -> Mux8/3
  Constant12/1 -> Mux8/2
  Demux3/1 -> Mux8/1
  Direction Cosine Matrix Body to Wind/1 -> Product1/1
  Product1/1 -> calc alpha_dot/3(Vw)
  "Incidence, Sideslip, & Airspeed"/1 -> Mux4/1
  "Incidence, Sideslip, & Airspeed"/3 -> Terminator/1
  Mux2/1 -> omega/1
  Mux1/1 -> omega_dot/1
  Mux6/1 -> Xe/1
  Product/1 -> Ve/1
  Mux8/1 -> Vb/1, "Incidence, Sideslip, & Airspeed"/1, [Vb]
  Rotation Angles to Direction Cosine Matrix/1 -> DCMbe/1, Transpose/1
  Constant5/1 -> Mux1/3
  Mux7/1 -> "alpha_dot, beta_dot"/1
  Memory1/1 -> Demux1/1
  AxAz/1 -> Memory1/1
  Memory2/1 -> Demux2/1
  XeZe/1 -> Memory2/1
  omega_y/1 -> Memory3/1
  Memory3/1 -> [q], Mux2/2
  uw/1 -> Memory4/1
  Memory4/1 -> Demux3/1
  dwdt/1 -> Memory5/1
  Memory5/1 -> Mux1/2
  theta/1 -> Memory6/1
  Memory6/1 -> Mux3/2

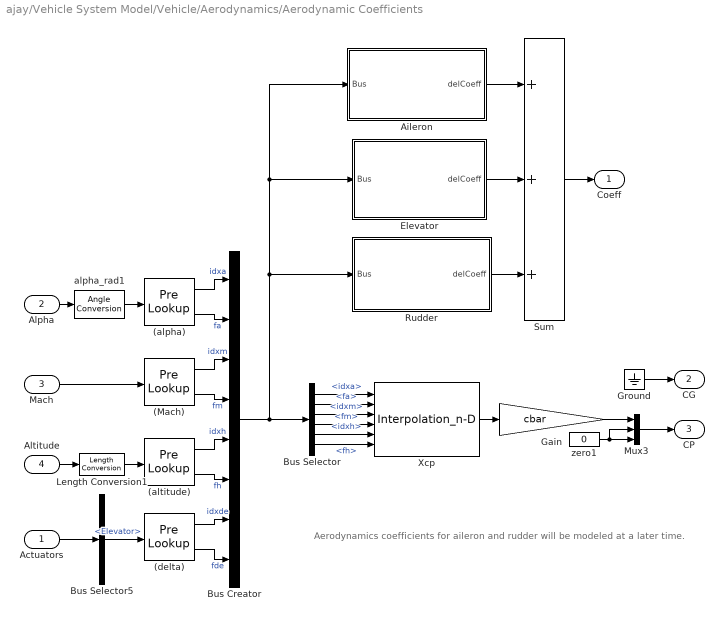
== system ajay/Vehicle System Model/Vehicle/Aerodynamics/Aerodynamic Coefficients ==
  note: Aerodynamics coefficients for aileron and rudder will be modeled at a later time.
  Actuators : Inport
  Alpha : Inport  Port=2
  Mach : Inport  Port=3
  Altitude : Inport  Port=4
  (Mach) : PreLookup  BreakpointsData=statdyn{1}.mach  BeginIndexSearchUsingPreviousIndexResult=on  ExtrapMethod=Linear  IndexDataTypeStr=int32  FractionDataTypeStr=double
  (alpha) : PreLookup  BreakpointsData=statdyn{1}.alpha  BeginIndexSearchUsingPreviousIndexResult=on  ExtrapMethod=Linear  IndexDataTypeStr=int32  FractionDataTypeStr=double
  (altitude) : PreLookup  BreakpointsData=statdyn{1}.alt  BeginIndexSearchUsingPreviousIndexResult=on  ExtrapMethod=Linear  IndexDataTypeStr=int32  FractionDataTypeStr=double
  (delta) : PreLookup  BreakpointsData=statdyn{1}.delta  BeginIndexSearchUsingPreviousIndexResult=on  ExtrapMethod=Linear  IndexDataTypeStr=int32  FractionDataTypeStr=double
  Aileron : Subsystem
  Bus Creator : BusCreator  Inputs=8
  Bus Selector : BusSelector  OutputSignals=idxa,fa,idxm,fm,idxh,fh
  Bus Selector5 : BusSelector  OutputSignals=Elevator
  Elevator : Subsystem
  Gain : Gain  Gain=cbar
  Ground : Ground
  Length Conversion1 : aerolibconvert2/Length Conversion  IU=m  OU=ft
  Mux3 : Mux  Inputs=3
  Rudder : Subsystem
  Sum : Sum  Inputs=3  InputSameDT=on  SaturateOnIntegerOverflow=on  OutDataTypeStr=Inherit: Same as first input
  Xcp : Interpolation_n-D  NumberOfTableDimensions=3  Table="permute(statdyn{1}.xcp,[1  2  3])"  OutDataTypeStr=double
      settings: InputPortMap=u0,u1,u2,u3,u4,u5
  alpha_rad1 : aerolibconvert2/Angle Conversion  IU=rad  OU=deg
  zero1 : Constant  Value=0
  Coeff : Outport  InitialOutput=0  VectorParamsAs1DForOutWhenUnconnected=off
  CG : Outport  Port=2  PortDimensions=3  InitialOutput=0  VectorParamsAs1DForOutWhenUnconnected=off
  CP : Outport  Port=3  PortDimensions=3  InitialOutput=0  VectorParamsAs1DForOutWhenUnconnected=off
  wires:
  Sum/1 -> Coeff/1
  Actuators/1 -> Bus Selector5/1
  Ground/1 -> CG/1
  Mux3/1 -> CP/1
  Xcp/1 -> Gain/1
  zero1/1 -> Mux3/2, Mux3/3
  Gain/1 -> Mux3/1
  (alpha)/2 -> Bus Creator/2  "fa"
  (Mach)/2 -> Bus Creator/4  "fm"
  (altitude)/2 -> Bus Creator/6  "fh"
  (altitude)/1 -> Bus Creator/5  "idxh"
  (Mach)/1 -> Bus Creator/3  "idxm"
  (alpha)/1 -> Bus Creator/1  "idxa"
  Bus Selector/1 -> Xcp/1  "<idxa>"
  Bus Selector/2 -> Xcp/2  "<fa>"
  Bus Selector/3 -> Xcp/3  "<idxm>"
  Bus Selector/4 -> Xcp/4  "<fm>"
  Bus Selector/5 -> Xcp/5  "<idxh>"
  Bus Selector/6 -> Xcp/6  "<fh>"
  Bus Creator/1 -> Bus Selector/1, Elevator/1(Bus), Aileron/1(Bus), Rudder/1(Bus)
  Mach/1 -> (Mach)/1
  Altitude/1 -> Length Conversion1/1
  Length Conversion1/1 -> (altitude)/1
  Alpha/1 -> alpha_rad1/1
  alpha_rad1/1 -> (alpha)/1
  Aileron/1(delCoeff) -> Sum/1
  Elevator/1(delCoeff) -> Sum/2
  Rudder/1(delCoeff) -> Sum/3
  (delta)/1 -> Bus Creator/7  "idxde"
  (delta)/2 -> Bus Creator/8  "fde"
  Bus Selector5/1 -> (delta)/1  "<Elevator>"

== system ajay/Vehicle System Model/Vehicle/Aerodynamics/DerivedConditions ==
  Speed of Sound : Inport
  Air Density : Inport  Port=2
  WindVelocity : Inport  Port=3  PortDimensions=3
  WindAngularRates : Inport  Port=4  PortDimensions=3
  Vb : Inport  Port=5  PortDimensions=3
  Dynamic Pressure : aerolibasang/Dynamic Pressure
  Mach Number : aerolibasang/Mach Number
  Sum2 : Sum  Inputs=|+-  InputSameDT=on  SaturateOnIntegerOverflow=on  OutDataTypeStr=Inherit: Same as first input
  Mach : Outport  VectorParamsAs1DForOutWhenUnconnected=off
  qbar : Outport  Port=2  InitialOutput=0  VectorParamsAs1DForOutWhenUnconnected=off
  "pqrWind " : Outport  Port=3  VectorParamsAs1DForOutWhenUnconnected=off
  wires:
  Speed of Sound/1 -> Mach Number/2
  Mach Number/1 -> Mach/1  "Mach"
  Air Density/1 -> Dynamic Pressure/2
  Dynamic Pressure/1 -> qbar/1  "qbar"
  WindAngularRates/1 -> "pqrWind "/1
  Vb/1 -> Sum2/1
  Sum2/1 -> Dynamic Pressure/1, Mach Number/1
  WindVelocity/1 -> Sum2/2

== system ajay/Vehicle System Model/Vehicle/3DOF to 6DOF/3DOF to 6DOF/calc alpha_dot ==
  alpha,beta : Inport
  Ab : Inport  Port=2
  Vw : Inport  Port=3
  Direction Cosine Matrix Body to Wind : aerolibtransform2/Direction Cosine Matrix Body to Wind
  Product1 : Product  Multiplication=Matrix(*)  InputSameDT=on  SaturateOnIntegerOverflow=on  OutDataTypeStr=Inherit: Same as first input
  Product2 : Product  Inputs=*/  InputSameDT=on  SaturateOnIntegerOverflow=on  OutDataTypeStr=Inherit: Same as first input
  Selector2 : Selector  IndexMode=Zero-based  InputPortWidth=3  IndexOptions=Index vector (dialog)  Indices=2  OutputSizes=1
  Selector3 : Selector  IndexMode=Zero-based  InputPortWidth=3  IndexOptions=Index vector (dialog)  Indices=0  OutputSizes=1
  alpha_dot : Outport  VectorParamsAs1DForOutWhenUnconnected=off
  wires:
  Direction Cosine Matrix Body to Wind/1 -> Product1/1
  Product1/1 -> Selector2/1
  Selector2/1 -> Product2/1
  Selector3/1 -> Product2/2
  alpha,beta/1 -> Direction Cosine Matrix Body to Wind/1
  Product2/1 -> alpha_dot/1
  Ab/1 -> Product1/2
  Vw/1 -> Selector3/1

== system ajay/Vehicle System Model/Vehicle/Aerodynamics/Aerodynamic Coefficients/Aileron ==
  note: Aerodynamics coefficients for aileron and rudder will be modeled at a later time when 6DOF model is developed.
  Bus : Inport
  Constant1 : Constant  Value=0
  Mux1 : Mux  Inputs=6
  Terminator : Terminator
  delCoeff : Outport  VectorParamsAs1DForOutWhenUnconnected=off
  wires:
  Mux1/1 -> delCoeff/1
  Constant1/1 -> Mux1/1, Mux1/2, Mux1/3, Mux1/4, Mux1/5, Mux1/6
  Bus/1 -> Terminator/1

== system ajay/Vehicle System Model/Vehicle/Aerodynamics/Aerodynamic Coefficients/Elevator ==
  Bus : Inport
  Bus Selector2 : BusSelector  OutputSignals=idxa,fa,idxm,fm,idxh,fh,idxde,fde
  Bus Selector3 : BusSelector  OutputSignals=idxde,fde,idxm,fm,idxh,fh
  Bus Selector5 : BusSelector  OutputSignals=idxde,fde,idxm,fm,idxh,fh
  Constant1 : Constant  Value=0
  DCDI : Interpolation_n-D  NumberOfTableDimensions=4  Table=permute(statdyn{1}.dcdi_sym,[1 3 4 2 ])  RemoveProtectionIndex=on
      settings: InputPortMap=u0,u1,u2,u3,u4,u5,u6,u7
  DCL : Interpolation_n-D  NumberOfTableDimensions=3  Table="permute(statdyn{1}.dcl_sym,[1  2  3])"  RemoveProtectionIndex=on
      settings: InputPortMap=u0,u1,u2,u3,u4,u5
  DCm : Interpolation_n-D  NumberOfTableDimensions=3  Table="permute(statdyn{1}.dcm_sym,[1  2  3])"  RemoveProtectionIndex=on
      settings: InputPortMap=u0,u1,u2,u3,u4,u5
  Mux1 : Mux  Inputs=6
  delCoeff : Outport  VectorParamsAs1DForOutWhenUnconnected=off
  wires:
  Mux1/1 -> delCoeff/1
  Bus/1 -> Bus Selector2/1, Bus Selector3/1, Bus Selector5/1
  DCDI/1 -> Mux1/1
  DCL/1 -> Mux1/3
  DCm/1 -> Mux1/5
  Constant1/1 -> Mux1/2, Mux1/4, Mux1/6
  Bus Selector2/1 -> DCDI/1  "<idxa>"
  Bus Selector2/2 -> DCDI/2  "<fa>"
  Bus Selector3/1 -> DCL/1  "<idxde>"
  Bus Selector3/2 -> DCL/2  "<fde>"
  Bus Selector5/1 -> DCm/1  "<idxde>"
  Bus Selector5/2 -> DCm/2  "<fde>"
  Bus Selector2/3 -> DCDI/3  "<idxm>"
  Bus Selector2/4 -> DCDI/4  "<fm>"
  Bus Selector2/5 -> DCDI/5  "<idxh>"
  Bus Selector2/6 -> DCDI/6  "<fh>"
  Bus Selector2/7 -> DCDI/7  "<idxde>"
  Bus Selector2/8 -> DCDI/8  "<fde>"
  Bus Selector3/3 -> DCL/3  "<idxm>"
  Bus Selector3/4 -> DCL/4  "<fm>"
  Bus Selector3/5 -> DCL/5  "<idxh>"
  Bus Selector3/6 -> DCL/6  "<fh>"
  Bus Selector5/3 -> DCm/3  "<idxm>"
  Bus Selector5/4 -> DCm/4  "<fm>"
  Bus Selector5/5 -> DCm/5  "<idxh>"
  Bus Selector5/6 -> DCm/6  "<fh>"

== system ajay/Vehicle System Model/Vehicle/Aerodynamics/Aerodynamic Coefficients/Rudder ==
  note: Aerodynamics coefficients for aileron and rudder will be modeled at a later time when 6DOF model is developed.
  Bus : Inport
  Constant1 : Constant  Value=0
  Mux1 : Mux  Inputs=6
  Terminator : Terminator
  delCoeff : Outport  VectorParamsAs1DForOutWhenUnconnected=off
  wires:
  Mux1/1 -> delCoeff/1
  Constant1/1 -> Mux1/6, Mux1/5, Mux1/4, Mux1/3, Mux1/2, Mux1/1
  Bus/1 -> Terminator/1
